simulink model "ThyristorWithContoller"  (R2018a)
settings: Solver=FixedStepDiscrete  StartTime=0.0  StopTime=50  RelTol=1e-3
libraries: powerlib x15
settings Model: Creator=enes_  LastModifiedBy=enes_

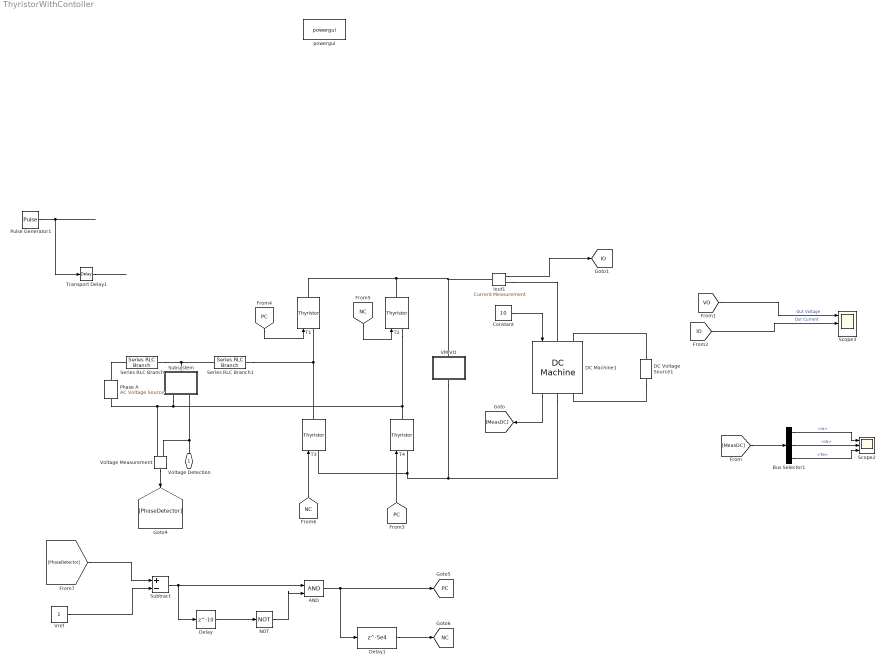
== system ThyristorWithContoller ==
  AND : Logic  IconShape=distinctive  AllPortsSameDT=off  OutDataTypeStr=boolean
  Bus Selector1 : BusSelector  OutputSignals=w,iA,Te
  Constant : Constant  Value=10
  DC Machine1 : powerlib/Machines/DC Machine  PresetModel=No  MechanicalLoad=Torque TL  FieldType=Wound  ShowDetailedParameters=on  MeasurementBus=on  RLa="[ 0.8  0.0125]"  RLf="[ 8260  6.4]"  Laf=5  MachineConstant=Torque constant (N.m/A)  Ke=1.8  Kt=1.8  J=0.3  Bm=0  Tf=0  w0=0  Ifinit=0  TsPowergui=0  TsBlock=-1
  DC Voltage Source1 : powerlib/Electrical Sources/DC Voltage Source  Amplitude=180  Measurements=None
  Delay : Delay  DelayLength=10
  Delay1 : Delay  DelayLength=5e4
  Iout1 : powerlib/Measurements/Current Measurement  PhasorSimulation=off  OutputType=Complex  PSBequivalent=0
  NOT : Logic  Operator=NOT  IconShape=distinctive  AllPortsSameDT=off  OutDataTypeStr=boolean
  Phase A : powerlib/Electrical Sources/AC Voltage Source  Amplitude=230*sqrt(2)  Phase=0  Frequency=50  SampleTime=0  Measurements=None  BusType=swing  Pref=10e3  Qref=0  Qmin=-inf  Qmax=+inf
  Pulse Generator1 : DiscretePulseGenerator  PulseType=Time based  Amplitude=5  Period=0.02  PulseWidth=5  PhaseDelay=(40*0.02)/360
  Scope2 : Scope  NumInputPorts=3
  Scope3 : Scope  NumInputPorts=3
  Series RLC Branch : powerlib/Elements/Series RLC Branch  LConnTagsString=__new0  RConnTagsString=__new0  BranchType=L  Resistance=1  Inductance=10e-9  SetiL0=off  InitialCurrent=0  Capacitance=1e-6  Setx0=off  InitialVoltage=0  Measurements=None
  Series RLC Branch1 : powerlib/Elements/Series RLC Branch  LConnTagsString=__new0  RConnTagsString=__new0  BranchType=L  Resistance=1  Inductance=10e-9  SetiL0=off  InitialCurrent=0  Capacitance=1e-6  Setx0=off  InitialVoltage=0  Measurements=None
  Subsystem : Subsystem
  Subtract : Sum  Inputs=+-
  T{1..4} (4 alike) : powerlib/Power Electronics/Thyristor  Ron=0.035  Lon=0  Vf=1.4  IC=0  Rs=68  Cs=100e-9  Measurements=off
  Transport Delay1 : TransportDelay  DelayTime=0.01
  VM VO : Subsystem
  Voltage Measurement : powerlib/Measurements/Voltage Measurement  PhasorSimulation=off  OutputType=Complex  PSBequivalent=0
  Vref : Constant
  powergui : powerlib/powergui  Priority=1  SimulationMode=Discrete  SampleTime=0.2e-6  frequency=60  Iterations=50  frequencyindice=0  Pbase=100e6  ErrMax=1e-4  UnitsV=kV  UnitsW=MW  buscounter=0  FunctionMessages=off  echomessages=off  EnableUseOfTLC=off  CurrentSourceSwitches=off  DisableSnubberDevices=off  DisableRonSwitches=off  DisableVfSwitches=off  DisplayEquations=off  SolverType=Tustin/Backward Euler (TBE)  Interpol=off  ExternalGateDelay=off  methode=off  Ts=100  x0status=blocks  SPID=off  SwTol=0  HookPort=off  RestoreLinks=warning  ResistiveCurrentMeasurement=off  Frange=[0:2:500]  Ylog=off  Xlog=on  ShowGrid=off  save=off  variable=ZData  structure=InputCurrent  ZoomFFT=off  StartTime=2.5  cycles=100  DisplayStyle=2  fundamental=50  FreqAxis=off  MaxFrequency=1000  frequencyindicesteady=1  RmsSteady=1  display=off
  Voltage Detection : PMIOPort  Side=Left
  tag scope: IO=global, NC=global, PC=global
  wires:
  DC Machine1/1 -> [MeasDC]
  [VO] -> Scope3/1  "Out Voltage"
  Iout1/1 -> [IO]
  [IO] -> Scope3/2  "Out Current"
  [PC] -> T1/1
  [PC] -> T4/1
  Pulse Generator1/1 -> Transport Delay1/1
  Transport Delay1/1 -> ?
  [NC] -> T2/1
  [NC] -> T3/1
  Constant/1 -> DC Machine1/1
  Bus Selector1/2 -> Scope2/2  "<iA>"
  Bus Selector1/1 -> Scope2/1  "<w>"
  [MeasDC] -> Bus Selector1/1
  Bus Selector1/3 -> Scope2/3  "<Te>"
  Voltage Measurement/1 -> [PhaseDetector]
  [PhaseDetector] -> Subtract/1
  Vref/1 -> Subtract/2
  Delay/1 -> NOT/1
  Subtract/1 -> Delay/1, AND/1
  NOT/1 -> AND/2
  AND/1 -> Delay1/1, [PC]
  Delay1/1 -> [NC]
  connections:
  T3/RConn1 -- Series RLC Branch1/RConn1 -- T1/LConn1
  DC Machine1/RConn1 -- VM VO/RConn1 -- T4/LConn1 -- T3/LConn1
  T1/RConn1 -- T2/RConn1 -- Iout1/LConn1 -- VM VO/LConn1
  Iout1/RConn1 -- DC Machine1/LConn1
  DC Voltage Source1/RConn1 -- DC Machine1/LConn2
  DC Voltage Source1/LConn1 -- DC Machine1/RConn2
  Phase A/RConn1 -- Series RLC Branch/LConn1
  Series RLC Branch/RConn1 -- Series RLC Branch1/LConn1 -- Subsystem/LConn1
  Phase A/LConn1 -- Voltage Measurement/LConn2 -- Subsystem/RConn1 -- T4/RConn1 -- T2/LConn1
  Voltage Detection/RConn1 -- Voltage Measurement/LConn1 -- Subsystem/RConn2

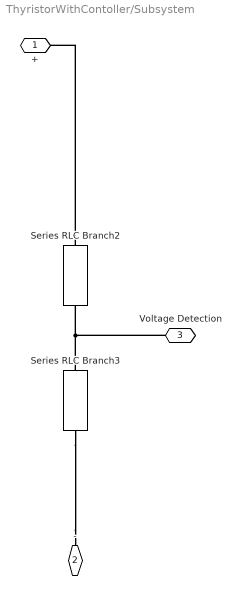
== system ThyristorWithContoller/Subsystem ==
  Series RLC Branch2 : powerlib/Elements/Series RLC Branch  LConnTagsString=__new0  RConnTagsString=__new0  BranchType=R  Resistance=64e3  Inductance=10e-9  SetiL0=off  InitialCurrent=0  Capacitance=1e-6  Setx0=off  InitialVoltage=0  Measurements=None
  Series RLC Branch3 : powerlib/Elements/Series RLC Branch  LConnTagsString=__new0  RConnTagsString=__new0  BranchType=R  Resistance=1e3  Inductance=10e-9  SetiL0=off  InitialCurrent=0  Capacitance=1e-6  Setx0=off  InitialVoltage=0  Measurements=None
  + : PMIOPort  Side=Left
  - : PMIOPort  Port=2  Side=Right
  Voltage Detection : PMIOPort  Port=3  Side=Right
  connections:
  Series RLC Branch3/LConn1 -- Series RLC Branch2/RConn1 -- Voltage Detection/RConn1
  Series RLC Branch2/LConn1 -- +/RConn1
  Series RLC Branch3/RConn1 -- -/RConn1

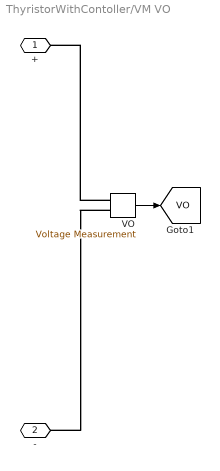
== system ThyristorWithContoller/VM VO ==
  VO : powerlib/Measurements/Voltage Measurement  PhasorSimulation=off  OutputType=Complex  PSBequivalent=0
  + : PMIOPort  Side=Left
  - : PMIOPort  Port=2  Side=Right
  tag scope: VO=global
  wires:
  VO/1 -> [VO]
  connections:
  VO/LConn2 -- -/RConn1
  VO/LConn1 -- +/RConn1
